simulink model "ClosedLoop_CqCsc"  (R2023b)
settings: Solver=VariableStepAuto  StartTime=0.0  StopTime=10.0  RelTol=1e-6
libraries: cstblocks x4
settings Model: Creator=bolee  LastModifiedBy=bolee

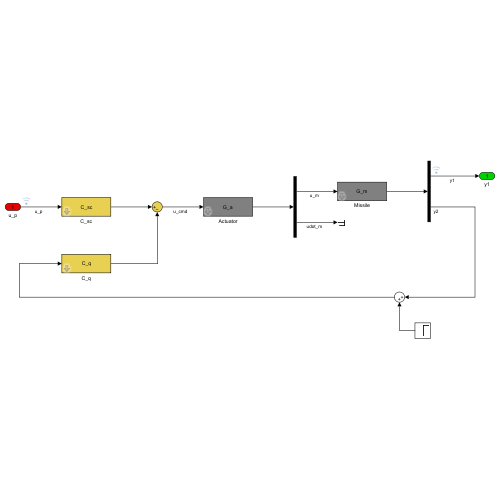
[thumbnail: Simulink's stored preview of the top-level diagram]
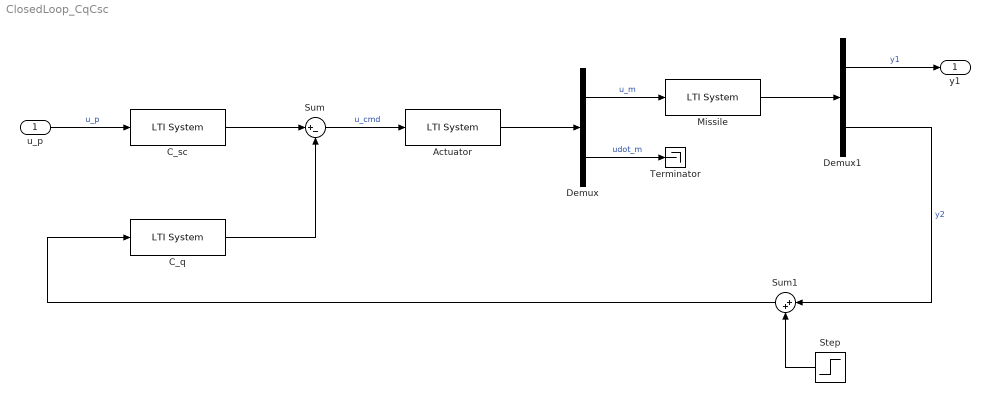
== system ClosedLoop_CqCsc ==
  u_p : Inport
  Actuator : cstblocks/LTI System  sys=G_a  IC=[]  PadeOrder=0
  C_q : cstblocks/LTI System  sys=C_q  IC=[]  PadeOrder=0
  C_sc : cstblocks/LTI System  sys=C_sc  IC=[]  PadeOrder=0
  Demux : Demux  Outputs=2
  Demux1 : Demux  Outputs=2
  Missile : cstblocks/LTI System  sys=G_m  IC=[]  PadeOrder=0
  Step : Step  SampleTime=0
  Sum : Sum  Inputs=|+-
  Sum1 : Sum  Inputs=|++
  Terminator : Terminator
  y1 : Outport
  wires:
  Actuator/1 -> Demux/1
  Sum/1 -> Actuator/1  "u_cmd"
  Demux/1 -> Missile/1  "u_m"
  Demux/2 -> Terminator/1  "udot_m"
  Missile/1 -> Demux1/1
  Demux1/1 -> y1/1  "y1"
  C_q/1 -> Sum/2
  C_sc/1 -> Sum/1
  u_p/1 -> C_sc/1  "u_p"
  Demux1/2 -> Sum1/1  "y2"
  Step/1 -> Sum1/2
  Sum1/1 -> C_q/1
